simulink model "gm_g"  (R2016b)
settings: Solver=FixedStepDiscrete  StartTime=0.0  StopTime=10.0  RelTol=1e-3
settings Model: Creator=hasee  LastModifiedBy=hasee
settings DataIOCC: LimitDataPoints=on  SaveOutput=off  SaveTime=off
settings OptimizationCC: BlockReduction=off  ConditionallyExecuteInputs=off  DefaultParameterBehavior=Inlined  LifeSpan=inf
settings DebuggingCC: AlgebraicLoopMsg=error  InheritedTsInSrcMsg=none  SingleTaskRateTransMsg=error  AllowSymbolicDim=off  StrictBusMsg=ErrorOnBusTreatedAsVector  SFUnexpectedBacktrackingDiag=warning  SFNoUnconditionalDefaultTransitionDiag=warning  SFExecutionAtInitializationDiag=none
settings HardwareCC: ProdBitPerPointer=32  ProdBitPerSizeT=32  ProdBitPerPtrDiffT=32  ProdLargestAtomicFloat=None  ProdIntDivRoundTo=Undefined  ProdEndianess=Unspecified  ProdWordSize=32  ProdHWDeviceType=ASIC/FPGA->ASIC/FPGA  ProdEqTarget=off
settings GRTTargetCC: TargetLangStandard=C89/C90 (ANSI)  GeneratePreprocessorConditionals=Disable all
settings ConfigComp: CovScope=ReferencedModels  CovMetricSettings=dw  CovHtmlReporting=on  CovSaveCumulativeToWorkspaceVar=on  CovSaveSingleToWorkspaceVar=on  CovExternalEMLEnable=off  CovSFcnEnable=off

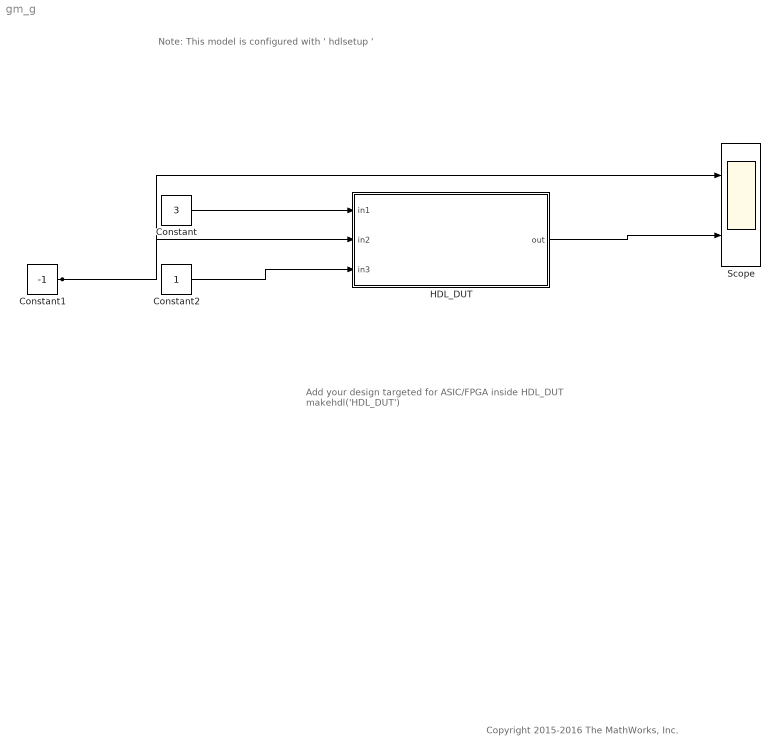
== system gm_g ==
  note: Copyright 2015-2016 The MathWorks, Inc.
  note: Add your design targeted for ASIC/FPGA inside HDL_DUT
      | makehdl('HDL_DUT')
  note: Note: This model is configured with ' hdlsetup '
  Constant : Constant  Value=3  OutDataTypeStr=int8  SampleTime=-1
  Constant1 : Constant  Value=-1  OutDataTypeStr=int8  SampleTime=-1
  Constant2 : Constant  OutDataTypeStr=boolean  SampleTime=-1
  HDL_DUT : Subsystem
  Scope : Scope  NumInputPorts=2
  wires:
  Constant/1 -> HDL_DUT/1(in1)
  Constant2/1 -> HDL_DUT/3(in3)
  Constant1/1 -> Scope/1, HDL_DUT/2(in2)
  HDL_DUT/1(out) -> Scope/2

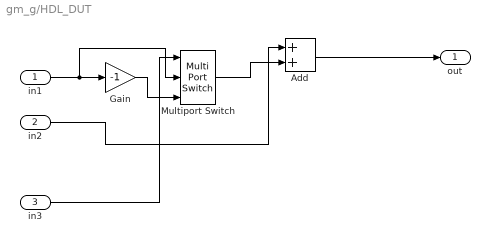
== system gm_g/HDL_DUT ==
  in1 : Inport
  in2 : Inport  Port=2
  in3 : Inport  Port=3  OutDataTypeStr=boolean
  Add : Sum  Inputs=2  AccumDataTypeStr=int8
  Gain : Gain  Gain=-1  OutDataTypeStr=int8
  Multiport Switch : MultiPortSwitch  DataPortOrder=Zero-based contiguous  Inputs=2  OutDataTypeStr=int8
  out : Outport
  wires:
  Add/1 -> out/1
  Multiport Switch/1 -> Add/2
  in2/1 -> Add/1
  Gain/1 -> Multiport Switch/3
  in3/1 -> Multiport Switch/1
  in1/1 -> Gain/1, Multiport Switch/2
